simulink subsystem "Wind_Model_2"  (R2026a)
settings: Solver=VariableStepAuto
values from neighbouring files (symbols this model uses):
  q = X(1:4)    [wind_fcn.m]
undefined symbols (not defined in the file or in its folder): constants6DoF, DiscIntNeverNeededParam, dt_SIM, F, Light, MIL, Wind_Covar, Wind_Gain, windMerid, windZonal
libraries: aerolibwind2 x1
settings Model: Creator=pplat  LastModifiedBy=alex2

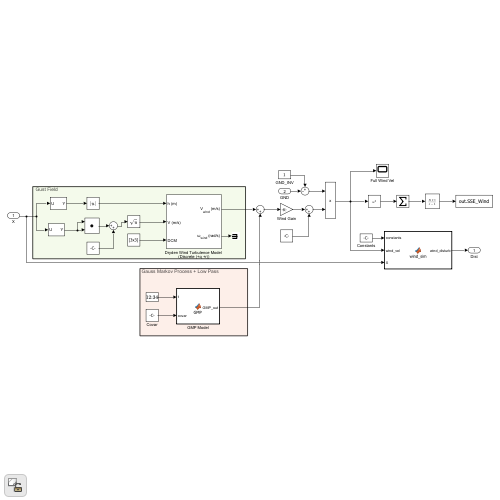
[thumbnail: Simulink's stored preview of the top-level diagram]
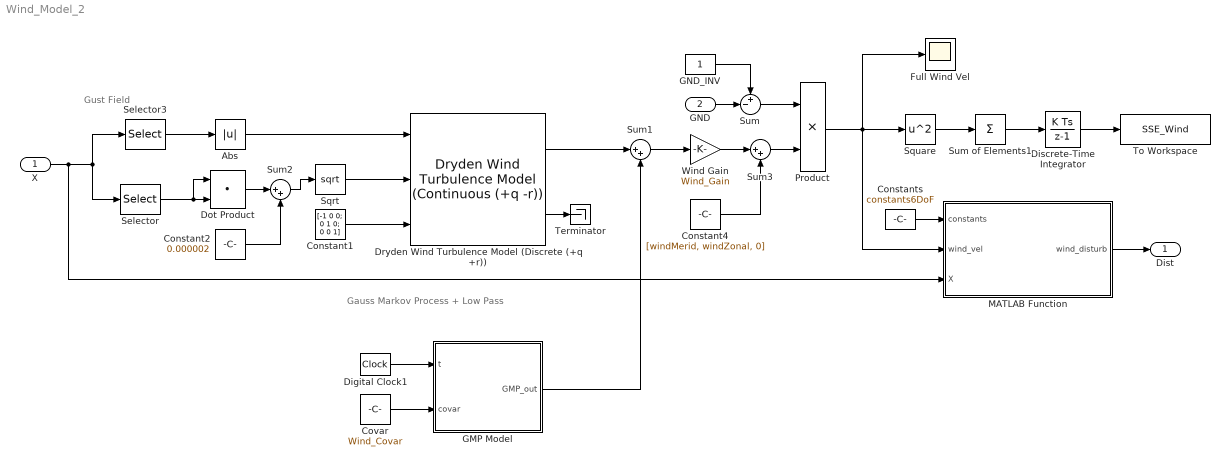
== system Wind_Model_2 ==
  note: Gust Field
  note: Gauss Markov Process + Low Pass
  X : Inport  PortDimensions=[15,1]
  GND : Inport  Port=2
  Abs : Abs  SaturateOnIntegerOverflow=off
  Constant1 : Constant  Value=[-1 0 0; 0 1 0; 0 0 1]
  Constant2 : Constant  Value=0.000002
  Constant4 : Constant  Value=[windMerid, windZonal, 0]
  Constants : Constant  Value=constants6DoF  OutDataTypeStr=Bus: Vehicle_Bus
  Covar : Constant  Value=Wind_Covar
  Digital Clock1 : DigitalClock  SampleTime=dt_SIM
  Discrete-Time Integrator : DiscreteIntegrator  InitialCondition=zeros(12,1)  SampleTime=-1  ICPrevOutput=DiscIntNeverNeededParam  ICPrevScaledInput=DiscIntNeverNeededParam
  Dot Product : DotProduct  OutDataTypeStr=Inherit: Inherit via internal rule
  Dryden Wind Turbulence Model (Discrete (+q +r)) : aerolibwind2/Dryden Wind Turbulence Model  (Continuous (+q -r))  units=Metric (MKS)  spec=MIL-F-8785C  model=Discrete Dryden (+q +r)  W20=15  Wdeg=0  TurbProb=10^-2 - Light  L_high=533.4  Wingspan=10  ts=0.1  Seed=[23341 23342 23343 23344]  T_on=on
      settings: LibrarySourceBlock=|
      | aerolibwind2/Dryden Wind Turbulence Model
      | (Discrete (+q +r))
  Full Wind Vel : Scope
      settings: ActiveDisplayYMinimum=-2.6741863438155993  ActiveDisplayYMaximum=6.3796567605614083  DataLoggingVariableName=ScopeData19
  GMP Model : MATLAB Function  TreatAsAtomicUnit=on
  GND_INV : Constant
  MATLAB Function : MATLAB Function  TreatAsAtomicUnit=on
  Product : Product
  Selector : Selector  IndexOptions=Index vector (dialog)  Indices=[8:10]  OutputSizes=1
  Selector3 : Selector  IndexOptions=Index vector (dialog)  Indices=7  OutputSizes=1
  Sqrt : Sqrt
  Square : Math  Operator=square
  Sum : Sum  Inputs=+-|
  Sum of Elements1 : Sum  Inputs=+
  Sum1 : Sum  Inputs=|++
  Sum2 : Sum  Inputs=|++
  Sum3 : Sum  Inputs=|++
  Terminator : Terminator
  To Workspace : ToWorkspace  VariableName=SSE_Wind  SampleTime=-1
      settings: MaxDataPoints=1
  Wind Gain : Gain  Gain=Wind_Gain
  Dist : Outport
  wires:
  GND_INV/1 -> Sum/1
  Covar/1 -> GMP Model/2(covar)
  GND/1 -> Sum/2
  MATLAB Function/1(wind_disturb) -> Dist/1
  Dot Product/1 -> Sum2/1
  GMP Model/1(GMP_out) -> Sum1/2
  Sum2/1 -> Sqrt/1
  Digital Clock1/1 -> GMP Model/1(t)
  Selector/1 -> Dot Product/2, Dot Product/1
  Constants/1 -> MATLAB Function/1(constants)
  Sum/1 -> Product/1
  Constant4/1 -> Sum3/2
  Constant2/1 -> Sum2/2
  Sum1/1 -> Wind Gain/1
  Wind Gain/1 -> Sum3/1
  Sum3/1 -> Product/2
  Abs/1 -> Dryden Wind Turbulence Model (Discrete (+q +r))/1
  Selector3/1 -> Abs/1
  X/1 -> Selector/1, Selector3/1, MATLAB Function/3(X)
  Constant1/1 -> Dryden Wind Turbulence Model (Discrete (+q +r))/3
  Sqrt/1 -> Dryden Wind Turbulence Model (Discrete (+q +r))/2
  Dryden Wind Turbulence Model (Discrete (+q +r))/1 -> Sum1/1
  Dryden Wind Turbulence Model (Discrete (+q +r))/2 -> Terminator/1
  Product/1 -> Full Wind Vel/1, MATLAB Function/2(wind_vel), Square/1
  Discrete-Time Integrator/1 -> To Workspace/1
  Square/1 -> Sum of Elements1/1
  Sum of Elements1/1 -> Discrete-Time Integrator/1

== matlab function Wind_Model_2/GMP Model ==
  data: t input; GMP_out output; covar input
function GMP_out = GMP(t, covar)

persistent errorval lastTime EMA
if isempty(errorval)
    errorval = 0;
    EMA = 0;
    lastTime = 0;  % Update last timestamp
end

dT = t - lastTime;

% First order Gauss Markov Process for additional disturbance
decay = 10;
beta = exp(-dT / decay);
errorval = beta * errorval + sqrt(1 - beta^2) * covar * randn;

% EMA Step to kill High Freq. Noise
EMA = ExpMovingAvg(errorval, EMA, 0.05);
GMP_out = EMA * ones(3,1);
lastTime = t;

== matlab function Wind_Model_2/MATLAB Function ==
  data: constants input; wind_vel input; X input; wind_disturb output
function wind_disturb = wind_sim(constants, wind_vel, X)

wind_disturb = wind_fcn(constants, wind_vel, X);
